simulink model "Campus_Power_System_updated"  (R2024a)
settings: Solver=daessc  StartTime=0.0  StopTime=1  RelTol=1e-3
libraries: spsThreePhaseVIMeasurementLib x57, spsThreePhaseTransformerTwoWindingsLib x56, spsThreePhaseSeriesRLCLoadLib x55, spsThreePhasePISectionLineLib x54, spsThreePhaseBreakerLib x9, spsCurrentMeasurementLib x3, spsMultimeterLib x1, spsThreePhaseSourceLib x1, spsThreePhaseFaultLib x1, sps_lib x1
(part 1 of 3)
settings Model: PacingRate=1000  Creator=dogba  LastModifiedBy=dogba

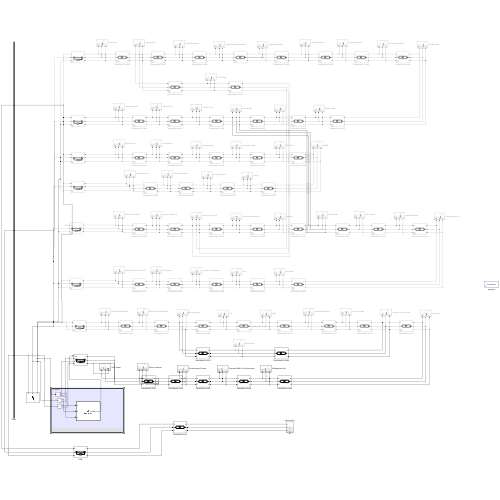
[thumbnail: Simulink's stored preview of the top-level diagram]
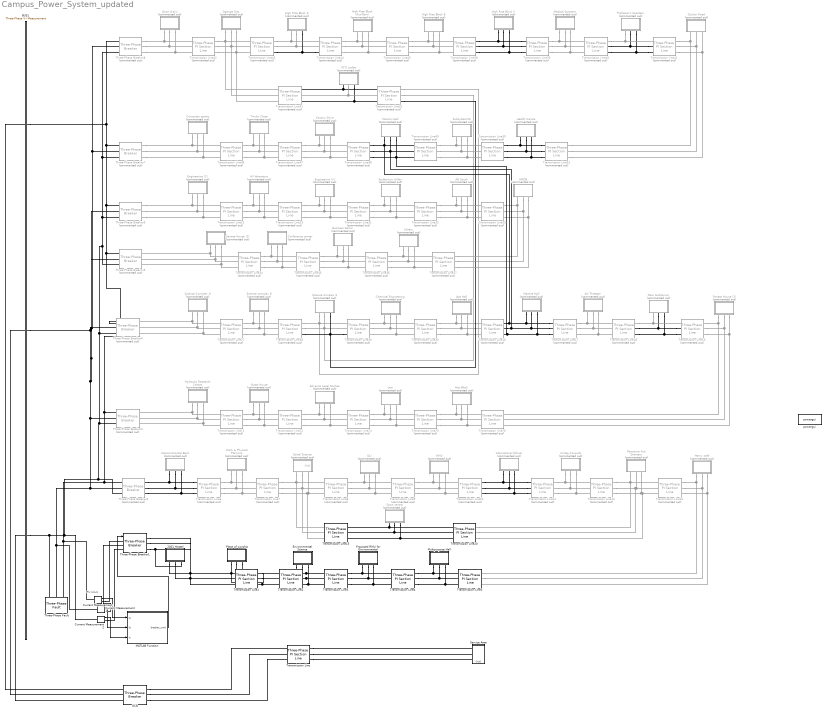
== system Campus_Power_System_updated ==
  note: Plc block
  2001 Hostel : Subsystem
  AG South : Subsystem  Commented=on
  Advance Legal Studies : Subsystem  Commented=on
  Alvan Ikoku : Subsystem  Commented=on
  Art Threater : Subsystem  Commented=on
  Arts Block : Subsystem  Commented=on
  Auditorium chiller : Subsystem  Commented=on
  BUS1 : spsThreePhaseVIMeasurementLib/Three-Phase V-I Measurement  VoltageMeasurement=no  SetLabelV=off  LabelV=Vabc  Vpu=off  VpuLL=off  CurrentMeasurement=no  SetLabelI=off  LabelI=Iabc  Ipu=off  Pbase=100e6  Vbase=500e3  OutputType=Complex  PhasorSimulation=off  PSBequivalent=0
  Business Admin : Subsystem  Commented=on
  Chemical Engineering : Subsystem  Commented=on
  Computer centre : Subsystem  Commented=on
  Conference center : Subsystem  Commented=on
  Current Measurement : spsCurrentMeasurementLib/Current Measurement  PhasorSimulation=off  OutputType=Complex  PSBequivalent=0
  Current Measurement1 : spsCurrentMeasurementLib/Current Measurement  PhasorSimulation=off  OutputType=Complex  PSBequivalent=0
  Current Measurement2 : spsCurrentMeasurementLib/Current Measurement  PhasorSimulation=off  OutputType=Complex  PSBequivalent=0
  DLI : Subsystem  Commented=on
  Engineering (1) : Subsystem  Commented=on
  Engineering (ii) : Subsystem  Commented=on
  Environmental Science : Subsystem
  Guest House : Subsystem  Commented=on
  HRDB : Subsystem  Commented=on
  HV laboratory : Subsystem  Commented=on
  Health Centre : Subsystem  Commented=on
  Henry cafe : Subsystem  Commented=on
  High Rise Block (Auxilliary) : Subsystem  Commented=on
  High Rise Block A : Subsystem  Commented=on
  High Rise Block B : Subsystem  Commented=on
  High Rise Block C : Subsystem  Commented=on
  Hydraulic Research Centre : Subsystem  Commented=on
  Intercontinental Bank : Subsystem  Commented=on
  International School : Subsystem  Commented=on
  Jaja Hall : Subsystem  Commented=on
  Kosoko Drive : Subsystem  Commented=on
  Law : Subsystem  Commented=on
  Library : Subsystem  Commented=on
  MATLAB Function : MATLAB Function  TreatAsAtomicUnit=on  SystemSampleTime=4e-4
  Main Auditorium : Subsystem  Commented=on
  Mareire Hall : Subsystem  Commented=on
  Medical Quarters : Subsystem  Commented=on
  Moremi Hall : Subsystem  Commented=on
  Multipurpose Hall : Subsystem
  OCB : spsThreePhaseBreakerLib/Three-Phase Breaker  InitialState=closed  SwitchA=on  SwitchB=on  SwitchC=on  SwitchTimes="[1/60  5/60]"  External=off  BreakerResistance=0.01  SnubberResistance=1e6  SnubberCapacitance=inf  Measurements=Breaker voltages and currents
  Ogenge Odo : Subsystem  Commented=on
  Ozukar Road : Subsystem  Commented=on
  Place of worship : Subsystem
  Professor's Quarters : Subsystem  Commented=on
  Proposed RMU for Environmental : Subsystem
  RMU : Subsystem  Commented=on
  Ransome Kuti Quarters : Subsystem  Commented=on
  Science Complex N : Subsystem  Commented=on
  Science Conplex S : Subsystem  Commented=on
  Science complex E : Subsystem  Commented=on
  Senate House (1) : Subsystem  Commented=on
  Senate House (2) : Subsystem  Commented=on
  Service Area : Subsystem
      settings: PortSchema="{\"entries\":[{\"content\":{\"sides\":[{\"content\":{},\"type\":\"ConnectorPlacement.EquallySpacedRectSide\",\"uuid\":\"a5d35126-4345-435f-8569-7a5f8796e1e8\"},{\"content\":{\"connectorIds\":[\"RConn1\",\"RConn2\",\"RConn3\"],\"side\":\"RIGHT\"},\"type\":\"ConnectorPlacement.EquallySpacedRectSide\",\"uuid\":\"f34b241a-7f4f-45ea-b4d4-6456543e546f\"},{\"content\":{\"side\":\"TOP\"},\"type\":\"ConnectorPlacement.EquallySpacedRectSide\",\"uuid\":\"c650f876-38c3-47f7-bb43-b6139a545593\"},{\"content\":{\"connectorIds\":[\"Out1\"],\"side\":\"BOTTOM\"},\"type\":\"ConnectorPlacement.EquallySpacedRectSide\",\"uuid\":\"fa4c8451-d781-46e6-9197-132e41a93a9a\"}]},\"type\":\"ConnectorPlacement.EquallySpacedConnector\",\"uuid\":\"f147ac36-e5db-452e-ba7f-0b8009a1ca04\"}],\"packageUris\":[\"http://schema.mathworks.com/mf0/Connector/R2020b\"],\"version\":\"1.0\"}"
  Social Science : Subsystem  Commented=on
      settings: PortSchema="{\"entries\":[{\"content\":{\"sides\":[{\"content\":{\"connectorIds\":[\"LConn1\",\"LConn2\",\"LConn3\"]},\"type\":\"ConnectorPlacement.EquallySpacedRectSide\",\"uuid\":\"e5269371-1ffa-4aff-ad38-defff3b9a2b6\"},{\"content\":{\"side\":\"RIGHT\"},\"type\":\"ConnectorPlacement.EquallySpacedRectSide\",\"uuid\":\"be72964e-51d9-4b4a-990d-c817bfc2f728\"},{\"content\":{\"side\":\"TOP\"},\"type\":\"ConnectorPlacement.EquallySpacedRectSide\",\"uuid\":\"61d5269b-ca21-4c37-9e34-ea928ee00b6f\"},{\"content\":{\"connectorIds\":[\"Out1\"],\"side\":\"BOTTOM\"},\"type\":\"ConnectorPlacement.EquallySpacedRectSide\",\"uuid\":\"d591f27b-b758-42fa-94ba-402f48fa72da\"}]},\"type\":\"ConnectorPlacement.EquallySpacedConnector\",\"uuid\":\"24f6a58e-2774-4bac-9805-d1b784781f4a\"}],\"packageUris\":[\"http://schema.mathworks.com/mf0/Connector/R2020b\"],\"version\":\"1.0\"}"
  Sport centre : Subsystem  Commented=on
  Subsystem53 : Subsystem  Commented=on
  Three-Phase Breaker1 : spsThreePhaseBreakerLib/Three-Phase Breaker  InitialState=closed  SwitchA=on  SwitchB=on  SwitchC=on  SwitchTimes="[1/60  5/60]"  External=on  BreakerResistance=0.01  SnubberResistance=1e6  SnubberCapacitance=inf  Measurements=Breaker voltages and currents
  Three-Phase Breaker{2..8} (7 alike) : spsThreePhaseBreakerLib/Three-Phase Breaker  Commented=on  InitialState=closed  SwitchA=on  SwitchB=on  SwitchC=on  SwitchTimes="[1/60  5/60]"  External=off  BreakerResistance=0.01  SnubberResistance=1e6  SnubberCapacitance=inf  Measurements=Breaker voltages and currents
  Three-Phase Fault : spsThreePhaseFaultLib/Three-Phase Fault  InitialStates=0  FaultA=off  FaultB=off  FaultC=on  GroundFault=on  SwitchTimes="[0.2  0.5]"  External=off  SwitchStatus=NaN  FaultResistance=0.001  GroundResistance=0.01  SnubberResistance=1e6  SnubberCapacitance=inf  Measurements=Fault voltages and currents
  Tinubu Close : Subsystem  Commented=on
  Transmission Line{,1..5,15,20} (8 alike) : spsThreePhasePISectionLineLib/Three-Phase PI Section Line  LConnTagsString=a|b|c  RConnTagsString=A|B|C  Length=0.5  Frequency=50  Resistances=[ 0.01273 0.3864]  Inductances="[ 0.9337e-3  4.1264e-3]"  Capacitances=[12.74e-9 7.751e-9]
  Transmission Line{6..14,16..19,21..53} (46 alike) : spsThreePhasePISectionLineLib/Three-Phase PI Section Line  Commented=on  LConnTagsString=a|b|c  RConnTagsString=A|B|C  Length=0.5  Frequency=50  Resistances=[ 0.01273 0.3864]  Inductances="[ 0.9337e-3  4.1264e-3]"  Capacitances=[12.74e-9 7.751e-9]
  Unilag Consults : Subsystem  Commented=on
  VC'S Lodge : Subsystem  Commented=on
  Work & Physical Planning : Subsystem  Commented=on
  powergui : sps_lib/powergui  Priority=1  SimulationMode=Continuous  SampleTime=50e-6  frequency=60  Iterations=50  frequencyindice=50  Pbase=100e6  ErrMax=1e-4  UnitsV=kV  UnitsW=MW  buscounter=0  FunctionMessages=off  echomessages=off  EnableUseOfTLC=off  CurrentSourceSwitches=off  DisableSnubberDevices=off  DisableRonSwitches=off  DisableVfSwitches=off  DisplayEquations=off  AutomaticDiscreteSolvers=off  SolverType=Tustin/Backward Euler (TBE)  Interpol=off  ExternalGateDelay=off  methode=off  Ts=100  x0status=blocks  SPID=on  SwTol=0  HookPort=off  NonlinearTolerance=1e-4  nMaxIteration=100  ContinueOnMaxIteration=off  RestoreLinks=warning  ResistiveCurrentMeasurement=off  Frange=[0:2:500]  Ylog=off  Xlog=on  ShowGrid=off  save=off  variable=ZData  structure=0  ZoomFFT=off  StartTime=0.0  cycles=1  DisplayStyle=1  fundamental=60  FreqAxis=off  MaxFrequency=1000  frequencyindicesteady=1  RmsSteady=1  display=off
  wires:
  MATLAB Function/1(breaker_cmd) -> Three-Phase Breaker1/1
  Current Measurement/1 -> MATLAB Function/1(Ia)
  Current Measurement1/1 -> MATLAB Function/2(Ib)
  Current Measurement2/1 -> MATLAB Function/3(Ic)
  connections:
  OCB/RConn1 -- Transmission Line/LConn1
  OCB/RConn2 -- Transmission Line/LConn2
  OCB/RConn3 -- Transmission Line/LConn3
  BUS1/RConn1 -- Three-Phase Breaker8/LConn1 -- Current Measurement/LConn1 -- Three-Phase Fault/LConn1 -- Three-Phase Breaker2/LConn1 -- Three-Phase Breaker3/LConn1 -- Three-Phase Breaker4/LConn1 -- Three-Phase Breaker5/LConn1 -- Three-Phase Breaker6/LConn1 -- Three-Phase Breaker7/LConn1
  BUS1/RConn2 -- Three-Phase Breaker4/LConn2 -- Three-Phase Breaker8/LConn2 -- Three-Phase Breaker7/LConn2 -- Three-Phase Breaker6/LConn2 -- Three-Phase Breaker5/LConn2 -- Current Measurement1/LConn1 -- Three-Phase Fault/LConn2 -- Three-Phase Breaker2/LConn2 -- Three-Phase Breaker3/LConn2
  BUS1/RConn3 -- Current Measurement2/LConn1 -- Three-Phase Breaker5/LConn3 -- Three-Phase Breaker8/LConn3 -- Three-Phase Breaker7/LConn3 -- Three-Phase Breaker6/LConn3 -- Three-Phase Breaker4/LConn3 -- Three-Phase Breaker3/LConn3 -- Three-Phase Breaker2/LConn3 -- Three-Phase Fault/LConn3
  BUS1/LConn1 -- OCB/LConn1
  BUS1/LConn2 -- OCB/LConn2
  BUS1/LConn3 -- OCB/LConn3
  Transmission Line/RConn3 -- Service Area/RConn3
  Transmission Line/RConn2 -- Service Area/RConn2
  Transmission Line/RConn1 -- Service Area/RConn1
  Three-Phase Breaker1/RConn1 -- Transmission Line1/LConn1 -- 2001 Hostel/LConn1
  Three-Phase Breaker1/RConn2 -- Transmission Line1/LConn2 -- 2001 Hostel/LConn2
  Three-Phase Breaker1/RConn3 -- 2001 Hostel/LConn3 -- Transmission Line1/LConn3
  Transmission Line1/RConn1 -- Place of worship/LConn1 -- Transmission Line2/LConn1
  Transmission Line1/RConn2 -- Place of worship/LConn2 -- Transmission Line2/LConn2
  Transmission Line1/RConn3 -- Transmission Line2/LConn3 -- Place of worship/LConn3
  Transmission Line2/RConn1 -- Environmental Science/LConn1 -- Transmission Line3/LConn1
  Transmission Line2/RConn2 -- Environmental Science/LConn2 -- Transmission Line3/LConn2
  Transmission Line2/RConn3 -- Environmental Science/LConn3 -- Transmission Line3/LConn3
  Transmission Line3/RConn1 -- Proposed RMU for Environmental/LConn1 -- Transmission Line4/LConn1
  Transmission Line3/RConn2 -- Transmission Line4/LConn2 -- Proposed RMU for Environmental/LConn2
  Transmission Line3/RConn3 -- Proposed RMU for Environmental/LConn3 -- Transmission Line4/LConn3
  Transmission Line4/RConn1 -- Multipurpose Hall/LConn1 -- Transmission Line5/LConn1
  Transmission Line4/RConn2 -- Multipurpose Hall/LConn2 -- Transmission Line5/LConn2
  Transmission Line4/RConn3 -- Multipurpose Hall/LConn3 -- Transmission Line5/LConn3
  Transmission Line7/RConn2 -- Transmission Line8/LConn2 -- Transmission Line15/LConn2 -- Social Science/LConn2
  Transmission Line6/RConn2 -- Work & Physical Planning/LConn2 -- Transmission Line7/LConn2
  Transmission Line6/RConn3 -- Work & Physical Planning/LConn3 -- Transmission Line7/LConn3
  Transmission Line6/LConn1 -- Three-Phase Breaker2/RConn1 -- Intercontinental Bank/LConn1
  Transmission Line6/RConn1 -- Work & Physical Planning/LConn1 -- Transmission Line7/LConn1
  Transmission Line6/LConn2 -- Three-Phase Breaker2/RConn2 -- Intercontinental Bank/LConn2
  Transmission Line9/RConn2 -- RMU/LConn2 -- Transmission Line10/LConn2
  Transmission Line9/RConn3 -- RMU/LConn3 -- Transmission Line10/LConn3
  Transmission Line8/RConn1 -- DLI/LConn1 -- Transmission Line9/LConn1
  Transmission Line8/RConn2 -- DLI/LConn2 -- Transmission Line9/LConn2
  Transmission Line9/RConn1 -- RMU/LConn1 -- Transmission Line10/LConn1
  Transmission Line7/RConn1 -- Transmission Line8/LConn1 -- Transmission Line15/LConn1 -- Social Science/LConn1
  Transmission Line7/RConn3 -- Transmission Line15/LConn3 -- Social Science/LConn3 -- Transmission Line8/LConn3
  Transmission Line8/RConn3 -- DLI/LConn3 -- Transmission Line9/LConn3
  Transmission Line6/LConn3 -- Three-Phase Breaker2/RConn3 -- Intercontinental Bank/LConn3
  Transmission Line12/RConn2 -- Unilag Consults/LConn2 -- Transmission Line13/LConn2
  Transmission Line13/RConn2 -- Transmission Line20/RConn2 -- Ransome Kuti Quarters/LConn2 -- Transmission Line14/LConn2
  Transmission Line14/RConn3 -- Transmission Line5/RConn3 -- Henry cafe/LConn3
  Transmission Line13/RConn3 -- Ransome Kuti Quarters/LConn3 -- Transmission Line20/RConn3 -- Transmission Line14/LConn3
  Transmission Line14/RConn2 -- Transmission Line5/RConn2 -- Henry cafe/LConn2
  Transmission Line14/RConn1 -- Transmission Line5/RConn1 -- Henry cafe/LConn1
  Transmission Line13/RConn1 -- Transmission Line20/RConn1 -- Transmission Line14/LConn1 -- Ransome Kuti Quarters/LConn1
  Transmission Line12/LConn3 -- Transmission Line10/RConn3 -- International School/LConn3
  Transmission Line12/RConn3 -- Unilag Consults/LConn3 -- Transmission Line13/LConn3
  Transmission Line12/RConn1 -- Unilag Consults/LConn1 -- Transmission Line13/LConn1
  Transmission Line12/LConn2 -- Transmission Line10/RConn2 -- International School/LConn2
  Transmission Line12/LConn1 -- Transmission Line10/RConn1 -- International School/LConn1
  Transmission Line20/LConn1 -- Sport centre/LConn1 -- Transmission Line15/RConn1
  Transmission Line20/LConn2 -- Transmission Line15/RConn2 -- Sport centre/LConn2
  Transmission Line20/LConn3 -- Sport centre/LConn3 -- Transmission Line15/RConn3
  Transmission Line22/RConn2 -- Advance Legal Studies/LConn2 -- Transmission Line24/LConn2
  Transmission Line25/RConn2 -- Arts Block/LConn2 -- Transmission Line26/LConn2
  Transmission Line27/RConn2 -- Science complex E/LConn2 -- Transmission Line28/LConn2
  Transmission Line29/RConn3 -- Chemical Engineering/LConn3 -- Transmission Line30/LConn3
  Transmission Line30/RConn1 -- Jaja Hall/LConn1 -- Transmission Line16/LConn1
  Transmission Line29/RConn1 -- Chemical Engineering/LConn1 -- Transmission Line30/LConn1
  Transmission Line22/RConn3 -- Advance Legal Studies/LConn3 -- Transmission Line24/LConn3
  Transmission Line30/RConn3 -- Jaja Hall/LConn3 -- Transmission Line16/LConn3
  Transmission Line30/RConn2 -- Jaja Hall/LConn2 -- Transmission Line16/LConn2
  Transmission Line27/RConn1 -- Science complex E/LConn1 -- Transmission Line28/LConn1
  Transmission Line27/RConn3 -- Science complex E/LConn3 -- Transmission Line28/LConn3
  Science Complex N/LConn2 -- Transmission Line27/LConn2 -- Three-Phase Breaker4/RConn2
  Hydraulic Research Centre/LConn1 -- Transmission Line11/LConn1 -- Three-Phase Breaker3/RConn1
  Science Complex N/LConn1 -- Transmission Line27/LConn1 -- Three-Phase Breaker4/RConn1
  Transmission Line11/RConn3 -- Guest House/LConn3 -- Transmission Line22/LConn3
  Transmission Line19/LConn3 -- Main Auditorium/LConn3 -- Transmission Line18/RConn3
  Transmission Line24/RConn3 -- Law/LConn3 -- Transmission Line25/LConn3
  Transmission Line19/LConn2 -- Transmission Line18/RConn2 -- Main Auditorium/LConn2
  Science Conplex S/LConn2 -- Transmission Line29/LConn2 -- Transmission Line52/RConn2 -- Transmission Line28/RConn2
  Transmission Line17/RConn2 -- Art Threater/LConn2 -- Transmission Line18/LConn2
  Transmission Line11/RConn1 -- Guest House/LConn1 -- Transmission Line22/LConn1
  Transmission Line28/RConn1 -- Science Conplex S/LConn1 -- Transmission Line52/RConn1 -- Transmission Line29/LConn1
  Hydraulic Research Centre/LConn2 -- Transmission Line11/LConn2 -- Three-Phase Breaker3/RConn2
  Transmission Line17/RConn3 -- Art Threater/LConn3 -- Transmission Line18/LConn3
  Transmission Line17/RConn1 -- Art Threater/LConn1 -- Transmission Line18/LConn1
  Transmission Line11/RConn2 -- Guest House/LConn2 -- Transmission Line22/LConn2
  Transmission Line29/LConn3 -- Transmission Line52/RConn3 -- Transmission Line28/RConn3 -- Science Conplex S/LConn3
  Transmission Line19/RConn3 -- Transmission Line26/RConn3 -- Senate House (2)/LConn3
  Science Complex N/LConn3 -- Transmission Line27/LConn3 -- Three-Phase Breaker4/RConn3
  Transmission Line19/RConn2 -- Transmission Line26/RConn2 -- Senate House (2)/LConn2
  Transmission Line19/RConn1 -- Transmission Line26/RConn1 -- Senate House (2)/LConn1
  Transmission Line29/RConn2 -- Chemical Engineering/LConn2 -- Transmission Line30/LConn2
  Transmission Line25/RConn3 -- Arts Block/LConn3 -- Transmission Line26/LConn3
  Transmission Line24/RConn1 -- Law/LConn1 -- Transmission Line25/LConn1
  Main Auditorium/LConn1 -- Transmission Line18/RConn1 -- Transmission Line19/LConn1
  Hydraulic Research Centre/LConn3 -- Transmission Line11/LConn3 -- Three-Phase Breaker3/RConn3
  Transmission Line24/RConn2 -- Law/LConn2 -- Transmission Line25/LConn2
  Transmission Line25/RConn1 -- Arts Block/LConn1 -- Transmission Line26/LConn1
  Transmission Line22/RConn1 -- Advance Legal Studies/LConn1 -- Transmission Line24/LConn1
  Transmission Line31/RConn1 -- Auditorium chiller/LConn1 -- Transmission Line32/LConn1
  Transmission Line32/RConn3 -- AG South/LConn3 -- Transmission Line33/LConn3
  Transmission Line31/RConn3 -- Auditorium chiller/LConn3 -- Transmission Line32/LConn3
  Transmission Line31/RConn2 -- Auditorium chiller/LConn2 -- Transmission Line32/LConn2
  Transmission Line21/RConn3 -- HV laboratory/LConn3 -- Transmission Line23/LConn3
  Transmission Line23/RConn3 -- Engineering (ii)/LConn3 -- Transmission Line31/LConn3
  Transmission Line23/RConn1 -- Engineering (ii)/LConn1 -- Transmission Line31/LConn1
  Transmission Line32/RConn2 -- AG South/LConn2 -- Transmission Line33/LConn2
  Engineering (1)/LConn2 -- Three-Phase Breaker6/RConn2 -- Transmission Line21/LConn2
  Transmission Line32/RConn1 -- AG South/LConn1 -- Transmission Line33/LConn1
  Transmission Line21/RConn2 -- HV laboratory/LConn2 -- Transmission Line23/LConn2
  Engineering (1)/LConn3 -- Three-Phase Breaker6/RConn3 -- Transmission Line21/LConn3
  Transmission Line23/RConn2 -- Engineering (ii)/LConn2 -- Transmission Line31/LConn2
  Transmission Line21/RConn1 -- HV laboratory/LConn1 -- Transmission Line23/LConn1
  Engineering (1)/LConn1 -- Three-Phase Breaker6/RConn1 -- Transmission Line21/LConn1
  Transmission Line36/RConn1 -- Library/LConn1 -- Transmission Line37/LConn1
  Transmission Line37/RConn3 -- Transmission Line33/RConn3 -- HRDB/LConn3
  Transmission Line36/RConn3 -- Library/LConn3 -- Transmission Line37/LConn3
  Transmission Line36/RConn2 -- Library/LConn2 -- Transmission Line37/LConn2
  Transmission Line34/RConn3 -- Conference center/LConn3 -- Transmission Line35/LConn3
  Transmission Line35/RConn3 -- Business Admin/LConn3 -- Transmission Line36/LConn3
  Transmission Line35/RConn1 -- Business Admin/LConn1 -- Transmission Line36/LConn1
  Transmission Line37/RConn2 -- Transmission Line33/RConn2 -- HRDB/LConn2
  Senate House (1)/LConn2 -- Transmission Line34/LConn2 -- Three-Phase Breaker5/RConn2
  Transmission Line37/RConn1 -- Transmission Line33/RConn1 -- HRDB/LConn1
  Transmission Line34/RConn2 -- Conference center/LConn2 -- Transmission Line35/LConn2
  Senate House (1)/LConn3 -- Transmission Line34/LConn3 -- Three-Phase Breaker5/RConn3
  Transmission Line35/RConn2 -- Business Admin/LConn2 -- Transmission Line36/LConn2
  Transmission Line34/RConn1 -- Conference center/LConn1 -- Transmission Line35/LConn1
  Senate House (1)/LConn1 -- Transmission Line34/LConn1 -- Three-Phase Breaker5/RConn1
  Transmission Line42/RConn2 -- Transmission Line43/LConn2 -- Transmission Line51/LConn2 -- Ogenge Odo/LConn2
  Transmission Line44/RConn3 -- High Rise Block (Auxilliary)/LConn3 -- Transmission Line45/LConn3
  Transmission Line45/RConn1 -- High Rise Block B/LConn1 -- Transmission Line38/LConn1
  Transmission Line42/RConn3 -- Transmission Line43/LConn3 -- Transmission Line51/LConn3 -- Ogenge Odo/LConn3
  Alvan Ikoku/LConn3 -- Three-Phase Breaker8/RConn3 -- Transmission Line42/LConn3
  Transmission Line44/RConn1 -- High Rise Block (Auxilliary)/LConn1 -- Transmission Line45/LConn1
  Transmission Line45/RConn3 -- High Rise Block B/LConn3 -- Transmission Line38/LConn3
  Transmission Line41/LConn3 -- Professor's Quarters/LConn3 -- Transmission Line40/RConn3
  Transmission Line45/RConn2 -- High Rise Block B/LConn2 -- Transmission Line38/LConn2
  Transmission Line41/RConn3 -- Transmission Line53/RConn3 -- Ozukar Road/LConn3
  Transmission Line41/LConn2 -- Transmission Line40/RConn2 -- Professor's Quarters/LConn2
  Transmission Line44/RConn2 -- High Rise Block (Auxilliary)/LConn2 -- Transmission Line45/LConn2
  High Rise Block A/LConn2 -- Transmission Line44/LConn2 -- Transmission Line43/RConn2
  Transmission Line39/RConn2 -- Medical Quarters/LConn2 -- Transmission Line40/LConn2
  Transmission Line39/LConn1 -- Transmission Line38/RConn1 -- High Rise Block C/LConn1
  Alvan Ikoku/LConn2 -- Transmission Line42/LConn2 -- Three-Phase Breaker8/RConn2
  Transmission Line39/RConn3 -- Medical Quarters/LConn3 -- Transmission Line40/LConn3
  Transmission Line44/LConn3 -- Transmission Line43/RConn3 -- High Rise Block A/LConn3
  Alvan Ikoku/LConn1 -- Transmission Line42/LConn1 -- Three-Phase Breaker8/RConn1
  Transmission Line42/RConn1 -- Transmission Line43/LConn1 -- Transmission Line51/LConn1 -- Ogenge Odo/LConn1
  Transmission Line39/LConn3 -- Transmission Line38/RConn3 -- High Rise Block C/LConn3
  Professor's Quarters/LConn1 -- Transmission Line40/RConn1 -- Transmission Line41/LConn1
  Transmission Line39/RConn1 -- Medical Quarters/LConn1 -- Transmission Line40/LConn1
  Transmission Line39/LConn2 -- Transmission Line38/RConn2 -- High Rise Block C/LConn2
  Transmission Line41/RConn1 -- Transmission Line53/RConn1 -- Ozukar Road/LConn1
  Transmission Line41/RConn2 -- Transmission Line53/RConn2 -- Ozukar Road/LConn2
  Transmission Line43/RConn1 -- Transmission Line44/LConn1 -- High Rise Block A/LConn1
  Transmission Line17/LConn1 -- Transmission Line16/RConn1 -- Moremi Hall/LConn1 -- Transmission Line48/RConn1 -- Transmission Line49/LConn1 -- Mareire Hall/LConn1
  Transmission Line49/RConn3 -- Subsystem53/LConn3 -- Transmission Line50/LConn3
  Transmission Line17/LConn3 -- Transmission Line16/RConn3 -- Moremi Hall/LConn3 -- Transmission Line48/RConn3 -- Transmission Line49/LConn3 -- Mareire Hall/LConn3
  Transmission Line17/LConn2 -- Transmission Line16/RConn2 -- Moremi Hall/LConn2 -- Transmission Line48/RConn2 -- Transmission Line49/LConn2 -- Mareire Hall/LConn2
  Transmission Line46/RConn3 -- Tinubu Close/LConn3 -- Transmission Line47/LConn3
  Transmission Line47/RConn3 -- Kosoko Drive/LConn3 -- Transmission Line48/LConn3
  Transmission Line47/RConn1 -- Kosoko Drive/LConn1 -- Transmission Line48/LConn1
  Transmission Line49/RConn2 -- Subsystem53/LConn2 -- Transmission Line50/LConn2
  Computer centre/LConn2 -- Three-Phase Breaker7/RConn2 -- Transmission Line46/LConn2
  Transmission Line49/RConn1 -- Subsystem53/LConn1 -- Transmission Line50/LConn1
  Transmission Line46/RConn2 -- Tinubu Close/LConn2 -- Transmission Line47/LConn2
  Computer centre/LConn3 -- Three-Phase Breaker7/RConn3 -- Transmission Line46/LConn3
  Transmission Line47/RConn2 -- Kosoko Drive/LConn2 -- Transmission Line48/LConn2
  Transmission Line46/RConn1 -- Tinubu Close/LConn1 -- Transmission Line47/LConn1
  Computer centre/LConn1 -- Three-Phase Breaker7/RConn1 -- Transmission Line46/LConn1
  Transmission Line51/RConn3 -- VC'S Lodge/LConn3 -- Transmission Line52/LConn3
  Transmission Line51/RConn1 -- Transmission Line52/LConn1 -- VC'S Lodge/LConn1
  Transmission Line52/LConn2 -- Transmission Line51/RConn2 -- VC'S Lodge/LConn2
  Transmission Line53/LConn1 -- Transmission Line50/RConn1 -- Health Centre/LConn1
  Transmission Line53/LConn2 -- Transmission Line50/RConn2 -- Health Centre/LConn2
  Transmission Line53/LConn3 -- Transmission Line50/RConn3 -- Health Centre/LConn3
  Current Measurement/RConn1 -- Three-Phase Breaker1/LConn1
  Three-Phase Breaker1/LConn2 -- Current Measurement1/RConn1
  Current Measurement2/RConn1 -- Three-Phase Breaker1/LConn3

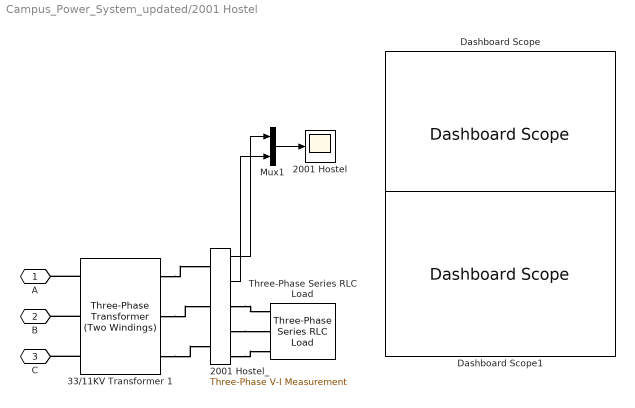
== system Campus_Power_System_updated/2001 Hostel ==
  2001 Hostel : Scope
  2001 Hostel_ : spsThreePhaseVIMeasurementLib/Three-Phase V-I Measurement  VoltageMeasurement=phase-to-ground  SetLabelV=off  LabelV=Vabc  Vpu=off  VpuLL=off  CurrentMeasurement=yes  SetLabelI=off  LabelI=Iabc  Ipu=off  Pbase=100e6  Vbase=500e3  OutputType=Complex  PhasorSimulation=off  PSBequivalent=0
  33/11KV Transformer 1 : spsThreePhaseTransformerTwoWindingsLib/Three-Phase Transformer (Two Windings)  Winding1Connection=Yg  Winding2Connection=Yg  CoreType=Three single-phase transformers  SetSaturation=off  Hysteresis=off  DataFile='hysteresis'  SetInitialFlux=off  Measurements=None  UNITS=pu  NominalPower=[ 250e6 , 50 ]  Winding1=[33e3 , 0.002 , 0.08 ]  Winding2=[ 11e3 , 0.002 , 0.08 ]  Rm=500  Lm=500  L0=0.5  Saturation=[ 0,0 ; 0.0024,1.2 ; 1.0,1.52 ]  InitialFluxes=[ 0.8 , -0.8 , 0.7 ]  BreakLoop=off  DiscreteSolver=Trapezoidal iterative  DataType=off  TransfoNumber=1
  Dashboard Scope : DashboardScope
  Dashboard Scope1 : DashboardScope
  Mux1 : Mux  Inputs=2
  Three-Phase Series RLC Load : spsThreePhaseSeriesRLCLoadLib/Three-Phase Series RLC Load  LConnTagsString=A|B|C  Configuration=Y (grounded)  NominalVoltage=220  Vabc=[1e3 1e3 1e3]  Vabcp=[1e3 1e3 1e3]  NominalFrequency=50  UnbalancedPower=off  ActivePower=140e3  InductivePower=100  CapacitivePower=100  Pabc=[10e3 9e3 11e3]  QLabc=[100 90 110]  QCabc=[100 90 110]  Pabcp=[10e3 9e3 11e3]  QLabcp=[100 90 110]  QCabcp=[100 90 110]  Measurements=None  LoadType=constant Z
  A : PMIOPort  Side=Left
  B : PMIOPort  Port=2  Side=Left
  C : PMIOPort  Port=3  Side=Left
  wires:
  2001 Hostel_/2 -> Mux1/2
  2001 Hostel_/1 -> Mux1/1
  Mux1/1 -> 2001 Hostel/1
  connections:
  33/11KV Transformer 1/RConn3 -- 2001 Hostel_/LConn3
  33/11KV Transformer 1/RConn1 -- 2001 Hostel_/LConn1
  2001 Hostel_/RConn2 -- Three-Phase Series RLC Load/LConn2
  2001 Hostel_/RConn3 -- Three-Phase Series RLC Load/LConn3
  33/11KV Transformer 1/RConn2 -- 2001 Hostel_/LConn2
  2001 Hostel_/RConn1 -- Three-Phase Series RLC Load/LConn1
  33/11KV Transformer 1/LConn1 -- A/RConn1
  33/11KV Transformer 1/LConn3 -- C/RConn1
  33/11KV Transformer 1/LConn2 -- B/RConn1

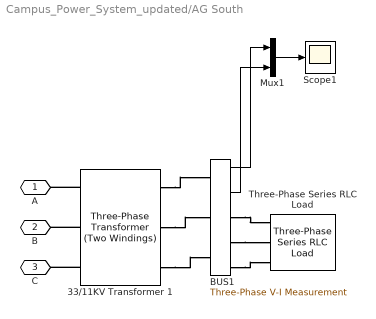
== system Campus_Power_System_updated/AG South ==
  33/11KV Transformer 1 : spsThreePhaseTransformerTwoWindingsLib/Three-Phase Transformer (Two Windings)  Winding1Connection=Yg  Winding2Connection=Yg  CoreType=Three single-phase transformers  SetSaturation=off  Hysteresis=off  DataFile='hysteresis'  SetInitialFlux=off  Measurements=None  UNITS=pu  NominalPower=[ 250e6 , 50 ]  Winding1=[33e3 , 0.002 , 0.08 ]  Winding2=[ 11e3 , 0.002 , 0.08 ]  Rm=500  Lm=500  L0=0.5  Saturation=[ 0,0 ; 0.0024,1.2 ; 1.0,1.52 ]  InitialFluxes=[ 0.8 , -0.8 , 0.7 ]  BreakLoop=off  DiscreteSolver=Trapezoidal iterative  DataType=off  TransfoNumber=1
  BUS1 : spsThreePhaseVIMeasurementLib/Three-Phase V-I Measurement  VoltageMeasurement=phase-to-ground  SetLabelV=off  LabelV=Vabc  Vpu=off  VpuLL=off  CurrentMeasurement=yes  SetLabelI=off  LabelI=Iabc  Ipu=off  Pbase=100e6  Vbase=500e3  OutputType=Complex  PhasorSimulation=off  PSBequivalent=0
  Mux1 : Mux  Inputs=2
  Scope1 : Scope
  Three-Phase Series RLC Load : spsThreePhaseSeriesRLCLoadLib/Three-Phase Series RLC Load  LConnTagsString=A|B|C  Configuration=Y (grounded)  NominalVoltage=1000  Vabc=[1e3 1e3 1e3]  Vabcp=[1e3 1e3 1e3]  NominalFrequency=60  UnbalancedPower=off  ActivePower=10e3  InductivePower=100  CapacitivePower=100  Pabc=[10e3 9e3 11e3]  QLabc=[100 90 110]  QCabc=[100 90 110]  Pabcp=[10e3 9e3 11e3]  QLabcp=[100 90 110]  QCabcp=[100 90 110]  Measurements=None  LoadType=constant Z
  A : PMIOPort  Side=Left
  B : PMIOPort  Port=2  Side=Left
  C : PMIOPort  Port=3  Side=Left
  wires:
  BUS1/2 -> Mux1/2
  BUS1/1 -> Mux1/1
  Mux1/1 -> Scope1/1
  connections:
  33/11KV Transformer 1/RConn3 -- BUS1/LConn3
  33/11KV Transformer 1/RConn1 -- BUS1/LConn1
  BUS1/RConn2 -- Three-Phase Series RLC Load/LConn2
  BUS1/RConn3 -- Three-Phase Series RLC Load/LConn3
  33/11KV Transformer 1/RConn2 -- BUS1/LConn2
  BUS1/RConn1 -- Three-Phase Series RLC Load/LConn1
  33/11KV Transformer 1/LConn1 -- A/RConn1
  33/11KV Transformer 1/LConn3 -- C/RConn1
  33/11KV Transformer 1/LConn2 -- B/RConn1

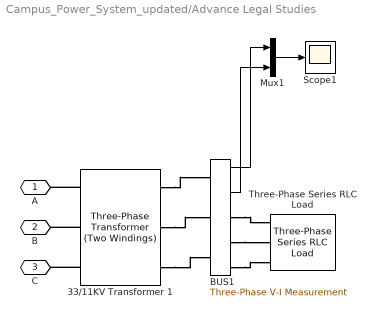
== system Campus_Power_System_updated/Advance Legal Studies ==
  33/11KV Transformer 1 : spsThreePhaseTransformerTwoWindingsLib/Three-Phase Transformer (Two Windings)  Winding1Connection=Yg  Winding2Connection=Yg  CoreType=Three single-phase transformers  SetSaturation=off  Hysteresis=off  DataFile='hysteresis'  SetInitialFlux=off  Measurements=None  UNITS=pu  NominalPower=[ 250e6 , 50 ]  Winding1=[33e3 , 0.002 , 0.08 ]  Winding2=[ 11e3 , 0.002 , 0.08 ]  Rm=500  Lm=500  L0=0.5  Saturation=[ 0,0 ; 0.0024,1.2 ; 1.0,1.52 ]  InitialFluxes=[ 0.8 , -0.8 , 0.7 ]  BreakLoop=off  DiscreteSolver=Trapezoidal iterative  DataType=off  TransfoNumber=1
  BUS1 : spsThreePhaseVIMeasurementLib/Three-Phase V-I Measurement  VoltageMeasurement=phase-to-ground  SetLabelV=off  LabelV=Vabc  Vpu=off  VpuLL=off  CurrentMeasurement=yes  SetLabelI=off  LabelI=Iabc  Ipu=off  Pbase=100e6  Vbase=500e3  OutputType=Complex  PhasorSimulation=off  PSBequivalent=0
  Mux1 : Mux  Inputs=2
  Scope1 : Scope
  Three-Phase Series RLC Load : spsThreePhaseSeriesRLCLoadLib/Three-Phase Series RLC Load  LConnTagsString=A|B|C  Configuration=Y (grounded)  NominalVoltage=1000  Vabc=[1e3 1e3 1e3]  Vabcp=[1e3 1e3 1e3]  NominalFrequency=60  UnbalancedPower=off  ActivePower=10e3  InductivePower=100  CapacitivePower=100  Pabc=[10e3 9e3 11e3]  QLabc=[100 90 110]  QCabc=[100 90 110]  Pabcp=[10e3 9e3 11e3]  QLabcp=[100 90 110]  QCabcp=[100 90 110]  Measurements=None  LoadType=constant Z
  A : PMIOPort  Side=Left
  B : PMIOPort  Port=2  Side=Left
  C : PMIOPort  Port=3  Side=Left
  wires:
  BUS1/2 -> Mux1/2
  BUS1/1 -> Mux1/1
  Mux1/1 -> Scope1/1
  connections:
  33/11KV Transformer 1/RConn3 -- BUS1/LConn3
  33/11KV Transformer 1/RConn1 -- BUS1/LConn1
  BUS1/RConn2 -- Three-Phase Series RLC Load/LConn2
  BUS1/RConn3 -- Three-Phase Series RLC Load/LConn3
  33/11KV Transformer 1/RConn2 -- BUS1/LConn2
  BUS1/RConn1 -- Three-Phase Series RLC Load/LConn1
  33/11KV Transformer 1/LConn1 -- A/RConn1
  33/11KV Transformer 1/LConn3 -- C/RConn1
  33/11KV Transformer 1/LConn2 -- B/RConn1

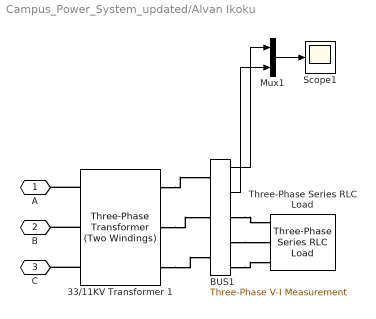
== system Campus_Power_System_updated/Alvan Ikoku ==
  33/11KV Transformer 1 : spsThreePhaseTransformerTwoWindingsLib/Three-Phase Transformer (Two Windings)  Winding1Connection=Yg  Winding2Connection=Yg  CoreType=Three single-phase transformers  SetSaturation=off  Hysteresis=off  DataFile='hysteresis'  SetInitialFlux=off  Measurements=None  UNITS=pu  NominalPower=[ 250e6 , 50 ]  Winding1=[33e3 , 0.002 , 0.08 ]  Winding2=[ 11e3 , 0.002 , 0.08 ]  Rm=500  Lm=500  L0=0.5  Saturation=[ 0,0 ; 0.0024,1.2 ; 1.0,1.52 ]  InitialFluxes=[ 0.8 , -0.8 , 0.7 ]  BreakLoop=off  DiscreteSolver=Trapezoidal iterative  DataType=off  TransfoNumber=1
  BUS1 : spsThreePhaseVIMeasurementLib/Three-Phase V-I Measurement  VoltageMeasurement=phase-to-ground  SetLabelV=off  LabelV=Vabc  Vpu=off  VpuLL=off  CurrentMeasurement=yes  SetLabelI=off  LabelI=Iabc  Ipu=off  Pbase=100e6  Vbase=500e3  OutputType=Complex  PhasorSimulation=off  PSBequivalent=0
  Mux1 : Mux  Inputs=2
  Scope1 : Scope
  Three-Phase Series RLC Load : spsThreePhaseSeriesRLCLoadLib/Three-Phase Series RLC Load  LConnTagsString=A|B|C  Configuration=Y (grounded)  NominalVoltage=1000  Vabc=[1e3 1e3 1e3]  Vabcp=[1e3 1e3 1e3]  NominalFrequency=60  UnbalancedPower=off  ActivePower=10e3  InductivePower=100  CapacitivePower=100  Pabc=[10e3 9e3 11e3]  QLabc=[100 90 110]  QCabc=[100 90 110]  Pabcp=[10e3 9e3 11e3]  QLabcp=[100 90 110]  QCabcp=[100 90 110]  Measurements=None  LoadType=constant Z
  A : PMIOPort  Side=Left
  B : PMIOPort  Port=2  Side=Left
  C : PMIOPort  Port=3  Side=Left
  wires:
  BUS1/2 -> Mux1/2
  BUS1/1 -> Mux1/1
  Mux1/1 -> Scope1/1
  connections:
  33/11KV Transformer 1/RConn3 -- BUS1/LConn3
  33/11KV Transformer 1/RConn1 -- BUS1/LConn1
  BUS1/RConn2 -- Three-Phase Series RLC Load/LConn2
  BUS1/RConn3 -- Three-Phase Series RLC Load/LConn3
  33/11KV Transformer 1/RConn2 -- BUS1/LConn2
  BUS1/RConn1 -- Three-Phase Series RLC Load/LConn1
  33/11KV Transformer 1/LConn1 -- A/RConn1
  33/11KV Transformer 1/LConn3 -- C/RConn1
  33/11KV Transformer 1/LConn2 -- B/RConn1

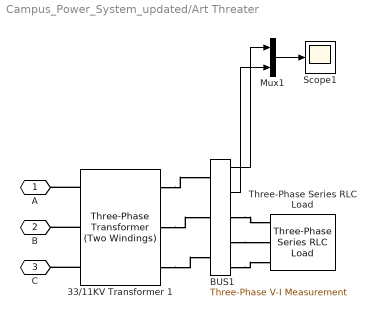
== system Campus_Power_System_updated/Art Threater ==
  33/11KV Transformer 1 : spsThreePhaseTransformerTwoWindingsLib/Three-Phase Transformer (Two Windings)  Winding1Connection=Yg  Winding2Connection=Yg  CoreType=Three single-phase transformers  SetSaturation=off  Hysteresis=off  DataFile='hysteresis'  SetInitialFlux=off  Measurements=None  UNITS=pu  NominalPower=[ 250e6 , 50 ]  Winding1=[33e3 , 0.002 , 0.08 ]  Winding2=[ 11e3 , 0.002 , 0.08 ]  Rm=500  Lm=500  L0=0.5  Saturation=[ 0,0 ; 0.0024,1.2 ; 1.0,1.52 ]  InitialFluxes=[ 0.8 , -0.8 , 0.7 ]  BreakLoop=off  DiscreteSolver=Trapezoidal iterative  DataType=off  TransfoNumber=1
  BUS1 : spsThreePhaseVIMeasurementLib/Three-Phase V-I Measurement  VoltageMeasurement=phase-to-ground  SetLabelV=off  LabelV=Vabc  Vpu=off  VpuLL=off  CurrentMeasurement=yes  SetLabelI=off  LabelI=Iabc  Ipu=off  Pbase=100e6  Vbase=500e3  OutputType=Complex  PhasorSimulation=off  PSBequivalent=0
  Mux1 : Mux  Inputs=2
  Scope1 : Scope
  Three-Phase Series RLC Load : spsThreePhaseSeriesRLCLoadLib/Three-Phase Series RLC Load  LConnTagsString=A|B|C  Configuration=Y (grounded)  NominalVoltage=1000  Vabc=[1e3 1e3 1e3]  Vabcp=[1e3 1e3 1e3]  NominalFrequency=60  UnbalancedPower=off  ActivePower=10e3  InductivePower=100  CapacitivePower=100  Pabc=[10e3 9e3 11e3]  QLabc=[100 90 110]  QCabc=[100 90 110]  Pabcp=[10e3 9e3 11e3]  QLabcp=[100 90 110]  QCabcp=[100 90 110]  Measurements=None  LoadType=constant Z
  A : PMIOPort  Side=Left
  B : PMIOPort  Port=2  Side=Left
  C : PMIOPort  Port=3  Side=Left
  wires:
  BUS1/2 -> Mux1/2
  BUS1/1 -> Mux1/1
  Mux1/1 -> Scope1/1
  connections:
  33/11KV Transformer 1/RConn3 -- BUS1/LConn3
  33/11KV Transformer 1/RConn1 -- BUS1/LConn1
  BUS1/RConn2 -- Three-Phase Series RLC Load/LConn2
  BUS1/RConn3 -- Three-Phase Series RLC Load/LConn3
  33/11KV Transformer 1/RConn2 -- BUS1/LConn2
  BUS1/RConn1 -- Three-Phase Series RLC Load/LConn1
  33/11KV Transformer 1/LConn1 -- A/RConn1
  33/11KV Transformer 1/LConn3 -- C/RConn1
  33/11KV Transformer 1/LConn2 -- B/RConn1

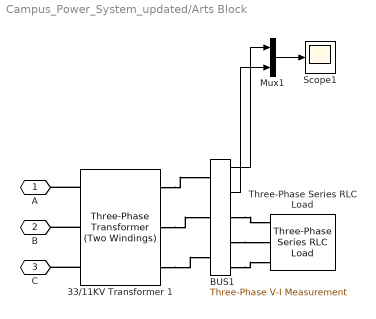
== system Campus_Power_System_updated/Arts Block ==
  33/11KV Transformer 1 : spsThreePhaseTransformerTwoWindingsLib/Three-Phase Transformer (Two Windings)  Winding1Connection=Yg  Winding2Connection=Yg  CoreType=Three single-phase transformers  SetSaturation=off  Hysteresis=off  DataFile='hysteresis'  SetInitialFlux=off  Measurements=None  UNITS=pu  NominalPower=[ 250e6 , 50 ]  Winding1=[33e3 , 0.002 , 0.08 ]  Winding2=[ 11e3 , 0.002 , 0.08 ]  Rm=500  Lm=500  L0=0.5  Saturation=[ 0,0 ; 0.0024,1.2 ; 1.0,1.52 ]  InitialFluxes=[ 0.8 , -0.8 , 0.7 ]  BreakLoop=off  DiscreteSolver=Trapezoidal iterative  DataType=off  TransfoNumber=1
  BUS1 : spsThreePhaseVIMeasurementLib/Three-Phase V-I Measurement  VoltageMeasurement=phase-to-ground  SetLabelV=off  LabelV=Vabc  Vpu=off  VpuLL=off  CurrentMeasurement=yes  SetLabelI=off  LabelI=Iabc  Ipu=off  Pbase=100e6  Vbase=500e3  OutputType=Complex  PhasorSimulation=off  PSBequivalent=0
  Mux1 : Mux  Inputs=2
  Scope1 : Scope
  Three-Phase Series RLC Load : spsThreePhaseSeriesRLCLoadLib/Three-Phase Series RLC Load  LConnTagsString=A|B|C  Configuration=Y (grounded)  NominalVoltage=1000  Vabc=[1e3 1e3 1e3]  Vabcp=[1e3 1e3 1e3]  NominalFrequency=60  UnbalancedPower=off  ActivePower=10e3  InductivePower=100  CapacitivePower=100  Pabc=[10e3 9e3 11e3]  QLabc=[100 90 110]  QCabc=[100 90 110]  Pabcp=[10e3 9e3 11e3]  QLabcp=[100 90 110]  QCabcp=[100 90 110]  Measurements=None  LoadType=constant Z
  A : PMIOPort  Side=Left
  B : PMIOPort  Port=2  Side=Left
  C : PMIOPort  Port=3  Side=Left
  wires:
  BUS1/2 -> Mux1/2
  BUS1/1 -> Mux1/1
  Mux1/1 -> Scope1/1
  connections:
  33/11KV Transformer 1/RConn3 -- BUS1/LConn3
  33/11KV Transformer 1/RConn1 -- BUS1/LConn1
  BUS1/RConn2 -- Three-Phase Series RLC Load/LConn2
  BUS1/RConn3 -- Three-Phase Series RLC Load/LConn3
  33/11KV Transformer 1/RConn2 -- BUS1/LConn2
  BUS1/RConn1 -- Three-Phase Series RLC Load/LConn1
  33/11KV Transformer 1/LConn1 -- A/RConn1
  33/11KV Transformer 1/LConn3 -- C/RConn1
  33/11KV Transformer 1/LConn2 -- B/RConn1

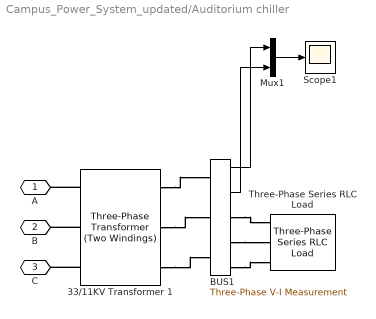
== system Campus_Power_System_updated/Auditorium chiller ==
  33/11KV Transformer 1 : spsThreePhaseTransformerTwoWindingsLib/Three-Phase Transformer (Two Windings)  Winding1Connection=Yg  Winding2Connection=Yg  CoreType=Three single-phase transformers  SetSaturation=off  Hysteresis=off  DataFile='hysteresis'  SetInitialFlux=off  Measurements=None  UNITS=pu  NominalPower=[ 250e6 , 50 ]  Winding1=[33e3 , 0.002 , 0.08 ]  Winding2=[ 11e3 , 0.002 , 0.08 ]  Rm=500  Lm=500  L0=0.5  Saturation=[ 0,0 ; 0.0024,1.2 ; 1.0,1.52 ]  InitialFluxes=[ 0.8 , -0.8 , 0.7 ]  BreakLoop=off  DiscreteSolver=Trapezoidal iterative  DataType=off  TransfoNumber=1
  BUS1 : spsThreePhaseVIMeasurementLib/Three-Phase V-I Measurement  VoltageMeasurement=phase-to-ground  SetLabelV=off  LabelV=Vabc  Vpu=off  VpuLL=off  CurrentMeasurement=yes  SetLabelI=off  LabelI=Iabc  Ipu=off  Pbase=100e6  Vbase=500e3  OutputType=Complex  PhasorSimulation=off  PSBequivalent=0
  Mux1 : Mux  Inputs=2
  Scope1 : Scope
  Three-Phase Series RLC Load : spsThreePhaseSeriesRLCLoadLib/Three-Phase Series RLC Load  LConnTagsString=A|B|C  Configuration=Y (grounded)  NominalVoltage=1000  Vabc=[1e3 1e3 1e3]  Vabcp=[1e3 1e3 1e3]  NominalFrequency=60  UnbalancedPower=off  ActivePower=10e3  InductivePower=100  CapacitivePower=100  Pabc=[10e3 9e3 11e3]  QLabc=[100 90 110]  QCabc=[100 90 110]  Pabcp=[10e3 9e3 11e3]  QLabcp=[100 90 110]  QCabcp=[100 90 110]  Measurements=None  LoadType=constant Z
  A : PMIOPort  Side=Left
  B : PMIOPort  Port=2  Side=Left
  C : PMIOPort  Port=3  Side=Left
  wires:
  BUS1/2 -> Mux1/2
  BUS1/1 -> Mux1/1
  Mux1/1 -> Scope1/1
  connections:
  33/11KV Transformer 1/RConn3 -- BUS1/LConn3
  33/11KV Transformer 1/RConn1 -- BUS1/LConn1
  BUS1/RConn2 -- Three-Phase Series RLC Load/LConn2
  BUS1/RConn3 -- Three-Phase Series RLC Load/LConn3
  33/11KV Transformer 1/RConn2 -- BUS1/LConn2
  BUS1/RConn1 -- Three-Phase Series RLC Load/LConn1
  33/11KV Transformer 1/LConn1 -- A/RConn1
  33/11KV Transformer 1/LConn3 -- C/RConn1
  33/11KV Transformer 1/LConn2 -- B/RConn1

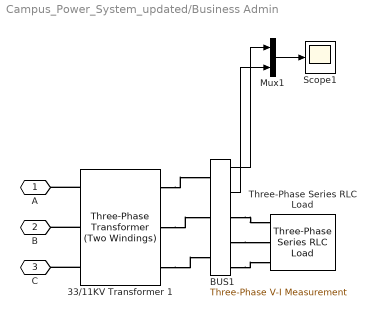
== system Campus_Power_System_updated/Business Admin ==
  33/11KV Transformer 1 : spsThreePhaseTransformerTwoWindingsLib/Three-Phase Transformer (Two Windings)  Winding1Connection=Yg  Winding2Connection=Yg  CoreType=Three single-phase transformers  SetSaturation=off  Hysteresis=off  DataFile='hysteresis'  SetInitialFlux=off  Measurements=None  UNITS=pu  NominalPower=[ 250e6 , 50 ]  Winding1=[33e3 , 0.002 , 0.08 ]  Winding2=[ 11e3 , 0.002 , 0.08 ]  Rm=500  Lm=500  L0=0.5  Saturation=[ 0,0 ; 0.0024,1.2 ; 1.0,1.52 ]  InitialFluxes=[ 0.8 , -0.8 , 0.7 ]  BreakLoop=off  DiscreteSolver=Trapezoidal iterative  DataType=off  TransfoNumber=1
  BUS1 : spsThreePhaseVIMeasurementLib/Three-Phase V-I Measurement  VoltageMeasurement=phase-to-ground  SetLabelV=off  LabelV=Vabc  Vpu=off  VpuLL=off  CurrentMeasurement=yes  SetLabelI=off  LabelI=Iabc  Ipu=off  Pbase=100e6  Vbase=500e3  OutputType=Complex  PhasorSimulation=off  PSBequivalent=0
  Mux1 : Mux  Inputs=2
  Scope1 : Scope
  Three-Phase Series RLC Load : spsThreePhaseSeriesRLCLoadLib/Three-Phase Series RLC Load  LConnTagsString=A|B|C  Configuration=Y (grounded)  NominalVoltage=1000  Vabc=[1e3 1e3 1e3]  Vabcp=[1e3 1e3 1e3]  NominalFrequency=60  UnbalancedPower=off  ActivePower=10e3  InductivePower=100  CapacitivePower=100  Pabc=[10e3 9e3 11e3]  QLabc=[100 90 110]  QCabc=[100 90 110]  Pabcp=[10e3 9e3 11e3]  QLabcp=[100 90 110]  QCabcp=[100 90 110]  Measurements=None  LoadType=constant Z
  A : PMIOPort  Side=Left
  B : PMIOPort  Port=2  Side=Left
  C : PMIOPort  Port=3  Side=Left
  wires:
  BUS1/2 -> Mux1/2
  BUS1/1 -> Mux1/1
  Mux1/1 -> Scope1/1
  connections:
  33/11KV Transformer 1/RConn3 -- BUS1/LConn3
  33/11KV Transformer 1/RConn1 -- BUS1/LConn1
  BUS1/RConn2 -- Three-Phase Series RLC Load/LConn2
  BUS1/RConn3 -- Three-Phase Series RLC Load/LConn3
  33/11KV Transformer 1/RConn2 -- BUS1/LConn2
  BUS1/RConn1 -- Three-Phase Series RLC Load/LConn1
  33/11KV Transformer 1/LConn1 -- A/RConn1
  33/11KV Transformer 1/LConn3 -- C/RConn1
  33/11KV Transformer 1/LConn2 -- B/RConn1

== system Campus_Power_System_updated/Chemical Engineering ==
  33/11KV Transformer 1 : spsThreePhaseTransformerTwoWindingsLib/Three-Phase Transformer (Two Windings)  Winding1Connection=Yg  Winding2Connection=Yg  CoreType=Three single-phase transformers  SetSaturation=off  Hysteresis=off  DataFile='hysteresis'  SetInitialFlux=off  Measurements=None  UNITS=pu  NominalPower=[ 250e6 , 50 ]  Winding1=[33e3 , 0.002 , 0.08 ]  Winding2=[ 11e3 , 0.002 , 0.08 ]  Rm=500  Lm=500  L0=0.5  Saturation=[ 0,0 ; 0.0024,1.2 ; 1.0,1.52 ]  InitialFluxes=[ 0.8 , -0.8 , 0.7 ]  BreakLoop=off  DiscreteSolver=Trapezoidal iterative  DataType=off  TransfoNumber=1
  BUS1 : spsThreePhaseVIMeasurementLib/Three-Phase V-I Measurement  VoltageMeasurement=phase-to-ground  SetLabelV=off  LabelV=Vabc  Vpu=off  VpuLL=off  CurrentMeasurement=yes  SetLabelI=off  LabelI=Iabc  Ipu=off  Pbase=100e6  Vbase=500e3  OutputType=Complex  PhasorSimulation=off  PSBequivalent=0
  Mux1 : Mux  Inputs=2
  Scope1 : Scope
  Three-Phase Series RLC Load : spsThreePhaseSeriesRLCLoadLib/Three-Phase Series RLC Load  LConnTagsString=A|B|C  Configuration=Y (grounded)  NominalVoltage=1000  Vabc=[1e3 1e3 1e3]  Vabcp=[1e3 1e3 1e3]  NominalFrequency=60  UnbalancedPower=off  ActivePower=10e3  InductivePower=100  CapacitivePower=100  Pabc=[10e3 9e3 11e3]  QLabc=[100 90 110]  QCabc=[100 90 110]  Pabcp=[10e3 9e3 11e3]  QLabcp=[100 90 110]  QCabcp=[100 90 110]  Measurements=None  LoadType=constant Z
  A : PMIOPort  Side=Left
  B : PMIOPort  Port=2  Side=Left
  C : PMIOPort  Port=3  Side=Left
  wires:
  BUS1/2 -> Mux1/2
  BUS1/1 -> Mux1/1
  Mux1/1 -> Scope1/1
  connections:
  33/11KV Transformer 1/RConn3 -- BUS1/LConn3
  33/11KV Transformer 1/RConn1 -- BUS1/LConn1
  BUS1/RConn2 -- Three-Phase Series RLC Load/LConn2
  BUS1/RConn3 -- Three-Phase Series RLC Load/LConn3
  33/11KV Transformer 1/RConn2 -- BUS1/LConn2
  BUS1/RConn1 -- Three-Phase Series RLC Load/LConn1
  33/11KV Transformer 1/LConn1 -- A/RConn1
  33/11KV Transformer 1/LConn3 -- C/RConn1
  33/11KV Transformer 1/LConn2 -- B/RConn1

== system Campus_Power_System_updated/Computer centre ==
  33/11KV Transformer 1 : spsThreePhaseTransformerTwoWindingsLib/Three-Phase Transformer (Two Windings)  Winding1Connection=Yg  Winding2Connection=Yg  CoreType=Three single-phase transformers  SetSaturation=off  Hysteresis=off  DataFile='hysteresis'  SetInitialFlux=off  Measurements=None  UNITS=pu  NominalPower=[ 250e6 , 50 ]  Winding1=[33e3 , 0.002 , 0.08 ]  Winding2=[ 11e3 , 0.002 , 0.08 ]  Rm=500  Lm=500  L0=0.5  Saturation=[ 0,0 ; 0.0024,1.2 ; 1.0,1.52 ]  InitialFluxes=[ 0.8 , -0.8 , 0.7 ]  BreakLoop=off  DiscreteSolver=Trapezoidal iterative  DataType=off  TransfoNumber=1
  BUS1 : spsThreePhaseVIMeasurementLib/Three-Phase V-I Measurement  VoltageMeasurement=phase-to-ground  SetLabelV=off  LabelV=Vabc  Vpu=off  VpuLL=off  CurrentMeasurement=yes  SetLabelI=off  LabelI=Iabc  Ipu=off  Pbase=100e6  Vbase=500e3  OutputType=Complex  PhasorSimulation=off  PSBequivalent=0
  Mux1 : Mux  Inputs=2
  Scope1 : Scope
  Three-Phase Series RLC Load : spsThreePhaseSeriesRLCLoadLib/Three-Phase Series RLC Load  LConnTagsString=A|B|C  Configuration=Y (grounded)  NominalVoltage=1000  Vabc=[1e3 1e3 1e3]  Vabcp=[1e3 1e3 1e3]  NominalFrequency=60  UnbalancedPower=off  ActivePower=10e3  InductivePower=100  CapacitivePower=100  Pabc=[10e3 9e3 11e3]  QLabc=[100 90 110]  QCabc=[100 90 110]  Pabcp=[10e3 9e3 11e3]  QLabcp=[100 90 110]  QCabcp=[100 90 110]  Measurements=None  LoadType=constant Z
  A : PMIOPort  Side=Left
  B : PMIOPort  Port=2  Side=Left
  C : PMIOPort  Port=3  Side=Left
  wires:
  BUS1/2 -> Mux1/2
  BUS1/1 -> Mux1/1
  Mux1/1 -> Scope1/1
  connections:
  33/11KV Transformer 1/RConn3 -- BUS1/LConn3
  33/11KV Transformer 1/RConn1 -- BUS1/LConn1
  BUS1/RConn2 -- Three-Phase Series RLC Load/LConn2
  BUS1/RConn3 -- Three-Phase Series RLC Load/LConn3
  33/11KV Transformer 1/RConn2 -- BUS1/LConn2
  BUS1/RConn1 -- Three-Phase Series RLC Load/LConn1
  33/11KV Transformer 1/LConn1 -- A/RConn1
  33/11KV Transformer 1/LConn3 -- C/RConn1
  33/11KV Transformer 1/LConn2 -- B/RConn1

== system Campus_Power_System_updated/Conference center ==
  33/11KV Transformer 1 : spsThreePhaseTransformerTwoWindingsLib/Three-Phase Transformer (Two Windings)  Winding1Connection=Yg  Winding2Connection=Yg  CoreType=Three single-phase transformers  SetSaturation=off  Hysteresis=off  DataFile='hysteresis'  SetInitialFlux=off  Measurements=None  UNITS=pu  NominalPower=[ 250e6 , 50 ]  Winding1=[33e3 , 0.002 , 0.08 ]  Winding2=[ 11e3 , 0.002 , 0.08 ]  Rm=500  Lm=500  L0=0.5  Saturation=[ 0,0 ; 0.0024,1.2 ; 1.0,1.52 ]  InitialFluxes=[ 0.8 , -0.8 , 0.7 ]  BreakLoop=off  DiscreteSolver=Trapezoidal iterative  DataType=off  TransfoNumber=1
  BUS1 : spsThreePhaseVIMeasurementLib/Three-Phase V-I Measurement  VoltageMeasurement=phase-to-ground  SetLabelV=off  LabelV=Vabc  Vpu=off  VpuLL=off  CurrentMeasurement=yes  SetLabelI=off  LabelI=Iabc  Ipu=off  Pbase=100e6  Vbase=500e3  OutputType=Complex  PhasorSimulation=off  PSBequivalent=0
  Mux1 : Mux  Inputs=2
  Scope1 : Scope
  Three-Phase Series RLC Load : spsThreePhaseSeriesRLCLoadLib/Three-Phase Series RLC Load  LConnTagsString=A|B|C  Configuration=Y (grounded)  NominalVoltage=1000  Vabc=[1e3 1e3 1e3]  Vabcp=[1e3 1e3 1e3]  NominalFrequency=60  UnbalancedPower=off  ActivePower=10e3  InductivePower=100  CapacitivePower=100  Pabc=[10e3 9e3 11e3]  QLabc=[100 90 110]  QCabc=[100 90 110]  Pabcp=[10e3 9e3 11e3]  QLabcp=[100 90 110]  QCabcp=[100 90 110]  Measurements=None  LoadType=constant Z
  A : PMIOPort  Side=Left
  B : PMIOPort  Port=2  Side=Left
  C : PMIOPort  Port=3  Side=Left
  wires:
  BUS1/2 -> Mux1/2
  BUS1/1 -> Mux1/1
  Mux1/1 -> Scope1/1
  connections:
  33/11KV Transformer 1/RConn3 -- BUS1/LConn3
  33/11KV Transformer 1/RConn1 -- BUS1/LConn1
  BUS1/RConn2 -- Three-Phase Series RLC Load/LConn2
  BUS1/RConn3 -- Three-Phase Series RLC Load/LConn3
  33/11KV Transformer 1/RConn2 -- BUS1/LConn2
  BUS1/RConn1 -- Three-Phase Series RLC Load/LConn1
  33/11KV Transformer 1/LConn1 -- A/RConn1
  33/11KV Transformer 1/LConn3 -- C/RConn1
  33/11KV Transformer 1/LConn2 -- B/RConn1

== system Campus_Power_System_updated/DLI ==
  33/11KV Transformer 1 : spsThreePhaseTransformerTwoWindingsLib/Three-Phase Transformer (Two Windings)  Winding1Connection=Yg  Winding2Connection=Yg  CoreType=Three single-phase transformers  SetSaturation=off  Hysteresis=off  DataFile='hysteresis'  SetInitialFlux=off  Measurements=None  UNITS=pu  NominalPower=[ 250e6 , 50 ]  Winding1=[33e3 , 0.002 , 0.08 ]  Winding2=[ 11e3 , 0.002 , 0.08 ]  Rm=500  Lm=500  L0=0.5  Saturation=[ 0,0 ; 0.0024,1.2 ; 1.0,1.52 ]  InitialFluxes=[ 0.8 , -0.8 , 0.7 ]  BreakLoop=off  DiscreteSolver=Trapezoidal iterative  DataType=off  TransfoNumber=1
  BUS1 : spsThreePhaseVIMeasurementLib/Three-Phase V-I Measurement  VoltageMeasurement=phase-to-ground  SetLabelV=off  LabelV=Vabc  Vpu=off  VpuLL=off  CurrentMeasurement=yes  SetLabelI=off  LabelI=Iabc  Ipu=off  Pbase=100e6  Vbase=500e3  OutputType=Complex  PhasorSimulation=off  PSBequivalent=0
  Mux1 : Mux  Inputs=2
  Scope1 : Scope
  Three-Phase Series RLC Load : spsThreePhaseSeriesRLCLoadLib/Three-Phase Series RLC Load  LConnTagsString=A|B|C  Configuration=Y (grounded)  NominalVoltage=1000  Vabc=[1e3 1e3 1e3]  Vabcp=[1e3 1e3 1e3]  NominalFrequency=60  UnbalancedPower=off  ActivePower=10e3  InductivePower=100  CapacitivePower=100  Pabc=[10e3 9e3 11e3]  QLabc=[100 90 110]  QCabc=[100 90 110]  Pabcp=[10e3 9e3 11e3]  QLabcp=[100 90 110]  QCabcp=[100 90 110]  Measurements=None  LoadType=constant Z
  A : PMIOPort  Side=Left
  B : PMIOPort  Port=2  Side=Left
  C : PMIOPort  Port=3  Side=Left
  wires:
  BUS1/2 -> Mux1/2
  BUS1/1 -> Mux1/1
  Mux1/1 -> Scope1/1
  connections:
  33/11KV Transformer 1/RConn3 -- BUS1/LConn3
  33/11KV Transformer 1/RConn1 -- BUS1/LConn1
  BUS1/RConn2 -- Three-Phase Series RLC Load/LConn2
  BUS1/RConn3 -- Three-Phase Series RLC Load/LConn3
  33/11KV Transformer 1/RConn2 -- BUS1/LConn2
  BUS1/RConn1 -- Three-Phase Series RLC Load/LConn1
  33/11KV Transformer 1/LConn1 -- A/RConn1
  33/11KV Transformer 1/LConn3 -- C/RConn1
  33/11KV Transformer 1/LConn2 -- B/RConn1
